simulink model "interpolation_nD_TestGen25"  (R2017b)
settings: Solver=FixedStepDiscrete  StartTime=0.0  StopTime=10.0  RelTol=1e-3
settings Model: Creator=ktrinh  LastModifiedBy=ktrinh
settings DebuggingCC: ParameterOverflowMsg=none

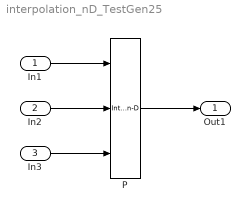
== system interpolation_nD_TestGen25 ==
  In1 : Inport  OutMin=0  OutMax=2  PortDimensions=1
  In2 : Inport  Port=2  OutMin=-0.5  OutMax=1.5
  In3 : Inport  Port=3  OutMin=0  OutMax=5
  P : Interpolation_n-D  Table=[26.287840591128 90.0127281190883 35.9555758743238 13.1167845673092 63.6452385982816;47.8051489656873 3.65209581369568 79.0361866798971 46.9731658019794 41.1033163980161]  InterpMethod=Nearest  ValidIndexMayReachLast=on  NumSelectionDims=1  OutDataTypeStr=uint8  InternalRulePriority=Speed  RndMeth=Round  SaturateOnIntegerOverflow=on  IntermediateResultsDataTypeStr=single
      settings: InputPortMap=u0,u1,u2
  Out1 : Outport
  wires:
  In1/1 -> P/1
  In2/1 -> P/2
  In3/1 -> P/3
  P/1 -> Out1/1
